simulink model "model_simple"  (R2016a)
settings: Solver=VariableStepAuto  StartTime=0.0  StopTime=100  RelTol=1e-3
settings Model: Creator=jani  LastModifiedBy=jani

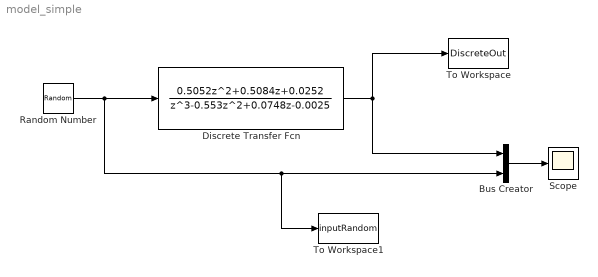
== system model_simple ==
  Bus Creator : BusCreator  Inputs=2
  Discrete Transfer Fcn : DiscreteTransferFcn  Numerator="[0       0.5052    0.5084    0.0252]"  Denominator="[1 -0.553    0.0748   -0.0025]"
  Random Number : RandomNumber  SampleTime=1
  Scope : Scope
  To Workspace : ToWorkspace  VariableName=DiscreteOut  SaveFormat=Timeseries  SampleTime=-1
  To Workspace1 : ToWorkspace  VariableName=inputRandom  SaveFormat=Timeseries  SampleTime=-1
  wires:
  Random Number/1 -> Bus Creator/2, To Workspace1/1, Discrete Transfer Fcn/1
  Discrete Transfer Fcn/1 -> Bus Creator/1, To Workspace/1
  Bus Creator/1 -> Scope/1
